simulink model "ex14busSGandPV_sim"  (R2014b)
settings: Solver=ode45  SolverMode=SingleTasking  StartTime=0.0  StopTime=8  MaxStep=0.0008  RelTol=0.0001
values from neighbouring files (symbols this model uses):
  Anf = full(Aksi)    [ex14busSGandPV.m]
  baseV = 1e3*mpcA.bus(1,BASE_KV)    [ex14busSGandPV.m]    (also in ex9busSG_data.mat = 345000; exDroopA.m = 1e3*mpc.bus(:,BASE_KV); exDroopB.m = 1e3*mpc.bus(:,BASE_KV); exLargeSysStability.m = 1e3*mpc.bus(:,BASE_KV))
  Bnf = full(Bksi)    [ex14busSGandPV.m]
  bus1_vd = 2^0.5*1e3    (= 1414.21356237)    [ex3busPV.m]    (also in exLongLinePV.m = 141421.356237)
  Cbus = [600e-6 ; 600e-6]    [ex14busSGandPV.m]    (also in exLongLinePV.m = 0.001)
  Cbus2 = (1e6*mpcC.bus(2,BS))/(ws*baseV^2)    [ex14busSGandPV.m]
  Cbus3 = (1e6*mpcC.bus(3,BS))/(ws*baseV^2)    [ex14busSGandPV.m]
  Cinv = Cinv_pu/(ws*baseZ)    [ex14busSGandPV.m]
  Cnf = full(Cksi)    [ex14busSGandPV.m]
  Dnf = full(Dksi)    [ex14busSGandPV.m]
  If_dc = 0.2*Prt./Ert    [ex14busSGandPV.m]    (also in ex7busLongLine.m = Prt./(60*Vf_dc); exDroopA.m = Prt./(60*Vf_dc); exDroopB.m = Prt./(60*Vf_dc); exSyncGenPVinv.m)
  Kd = KD_GAIN_CNST*J*ws    [ex14busSGandPV.m]    (also in ex2busStability.m = 24000; ex7busLongLine.m; ex9busSG.m; exDroopA.m)
  ki = [0.3 ; 0.3]    [ex14busSGandPV.m]    (also in exLongLinePV.m = 1e-05)
  kp = [1.3e-6 ; 1.3e-6]    [ex14busSGandPV.m]    (also in exLongLinePV.m = 1e-05)
  L0 = 0.1*Ld    [ex14busSGandPV.m]    (also in ex7busLongLine.m; exDroopA.m; exDroopB.m; exSyncGenPVinv.m)
  Laf = (2^0.5)*Ert./(ws*If_dc)    [ex14busSGandPV.m]    (also in ex7busLongLine.m; exDroopA.m; exDroopB.m; exSyncGenPVinv.m = (2^0.5)*5*Ert.^2./(ws*Prt))
  Lb2 = 2*Ld.*Lff - 3*Laf.^2    [ex14busSGandPV.m]    (also in ex7busLongLine.m; exDroopA.m; exDroopB.m; exSyncGenPVinv.m)
  Ld = 0.6*Lpu    [ex14busSGandPV.m]    (also in ex7busLongLine.m = 0.3*Lpu; exDroopA.m = 0.3*Lpu; exDroopB.m = 0.3*Lpu; exSyncGenPVinv.m)
  Lff = 2*Laf.^2./Ld    [ex14busSGandPV.m]    (also in ex7busLongLine.m; exDroopA.m; exDroopB.m; exSyncGenPVinv.m)
  Lq = Ld    [ex14busSGandPV.m]    (also in ex7busLongLine.m; exDroopA.m; exDroopB.m; exSyncGenPVinv.m)
  mpcE = runpf(mpcE)    [ex14busSGandPV.m]    (also in exDroopA.m)
  Nss = length(ssbus)    [ex14busSGandPV.m]
  PG = 2    [ex9busSG_data.mat]
  Pgm = 3*[40; 20]*1e6    [ex14busSGandPV.m]
  poles_2Jws = poles./(2*J*ws)    [ex14busSGandPV.m]    (also in ex2busStability.m = poles./(2*ws*J); ex7busLongLine.m; ex9busSG.m = poles./(2*ws*J); exDroopA.m)
  Pren = [10 ; 10]*1e6    [ex14busSGandPV.m]    (also in ex3busPV.m = 500; exLongLinePV.m = 5000000)
  PT = 16    [ex9busSG_data.mat]
  QG = 3    [ex9busSG_data.mat]
  QT = 17    [ex9busSG_data.mat]
  Ra = 0.05*Ert.^2./Prt    [ex14busSGandPV.m]    (also in ex7busLongLine.m = 0.01*Ert.^2./Prt; exDroopA.m = 0.01*Ert.^2./Prt; exDroopB.m = 0.01*Ert.^2./Prt; exSyncGenPVinv.m)
  Rf = Lff/1.2    [ex14busSGandPV.m]    (also in ex7busLongLine.m = Vf_dc./If_dc; exDroopA.m = Vf_dc./If_dc; exDroopB.m = Vf_dc./If_dc; exSyncGenPVinv.m)
  step_size_bus2 = 0    [ex14busSGandPV.m]
  step_size_bus3 = 0    [ex14busSGandPV.m]
  step_size_bus6 = 0    [ex14busSGandPV.m]
  step_size_bus8 = 0    [ex14busSGandPV.m]
  step_time_bus2 = 3    [ex14busSGandPV.m]
  step_time_bus3 = 3    [ex14busSGandPV.m]
  step_time_bus6 = 5    [ex14busSGandPV.m]
  step_time_bus8 = 5    [ex14busSGandPV.m]
  VA = 9    [ex9busSG_data.mat]
  Vbus_ref = [800 ; 800]    [ex14busSGandPV.m]    (also in exLongLinePV.m = 800)
  Vf_dc = If_dc.*Rf    [ex14busSGandPV.m]    (also in ex7busLongLine.m = 500 * ones(size(Ert)); exDroopA.m = 500 * ones(size(Ert)); exDroopB.m = 500 * ones(size(Ert)); exSyncGenPVinv.m)
  vinf_0 = 0    [ex14busSGandPV.m]    (also in ex7busLongLine.m; exDroopA.m; exSyncGenPVinv.m)
  vinf_d = (2^0.5)*mpcA.bus(1,VM)*baseV    [ex14busSGandPV.m]    (also in ex7busLongLine.m = 250457.221896; exDroopA.m = (2^0.5)*mpc.bus(1,VM)*baseV(1); exSyncGenPVinv.m = (2^0.5)*mpc.bus(1,VM)*baseV(1))
  vinf_q = 0    [ex14busSGandPV.m]    (also in ex7busLongLine.m; exDroopA.m; exSyncGenPVinv.m)
  vinit_dq0_bus2 = [real(vpp) ; imag(vpp) ; 0]    [ex14busSGandPV.m]
  vinit_dq0_bus3 = [real(vpp) ; imag(vpp) ; 0]    [ex14busSGandPV.m]
  vinit_dq0_bus6 = [real(vpp) ; imag(vpp) ; 0]    [ex14busSGandPV.m]
  vinit_dq0_bus8 = [real(vpp) ; imag(vpp) ; 0]    [ex14busSGandPV.m]
  VM = 8    [ex9busSG_data.mat]
  ws = 2*pi*50    (= 314.159265359)    [ex14busSGandPV.m]    (also in ex2busStability.m; ex3busPV.m; ex7busLongLine.m; ex9busSG.m)
libraries: simulink x2
(part 1 of 2)
settings Model: Creator=COPEC  LastModifiedBy=Juri
settings OptimizationCC: BlockReduction=off  BooleanDataType=off
settings DebuggingCC: SaveWithParameterizedLinksMsg=none  UnderspecifiedInitializationDetection=Classic  MergeDetectMultiDrivingBlocksExec=none  SignalResolutionControl=TryResolveAllWithWarning  SolverPrmCheckMsg=none  FrameProcessingCompatibilityMsg=error
settings HardwareCC: TargetUnknown=on

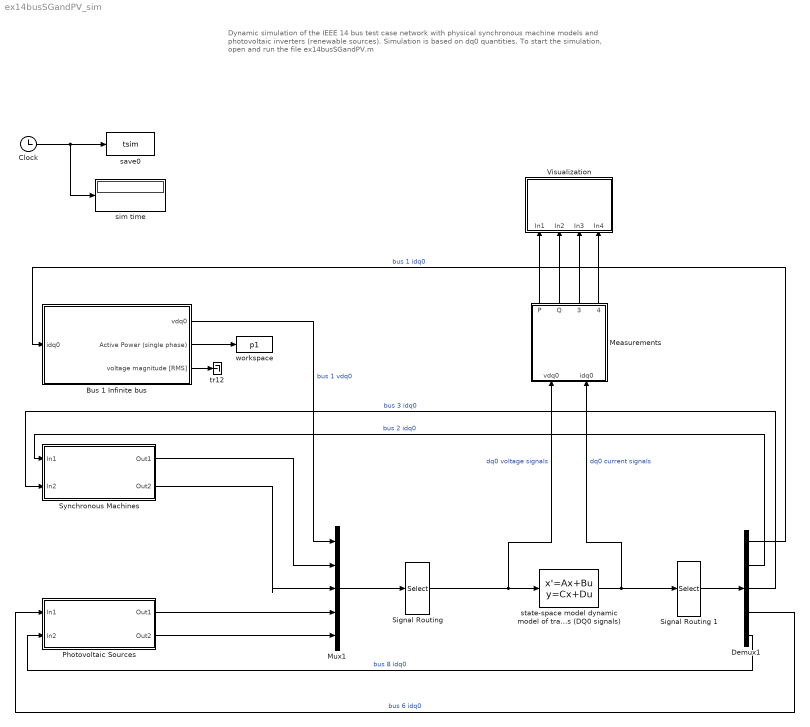
== system ex14busSGandPV_sim ==
  note: Dynamic simulation of the IEEE 14 bus test case network with physical synchronous machine models and photovoltaic inverters (renewable sources). Simulation is based on dq0 quantities.
      |
      | To start the simulation, open and run the file
      | ex14busSGandPV.m
  Bus 1 Infinite bus : Subsystem
  Clock : Clock
  Demux1 : Demux  Outputs=5
  Measurements : Subsystem
  Mux1 : Mux  Inputs=5
  Photovoltaic Sources : Subsystem
  "Signal Routing " : Selector  InputPortWidth=3*Nss  IndexOptions=Index vector (dialog)  Indices=units_to_net  OutputSizes=1
  Signal Routing 1 : Selector  InputPortWidth=3*Nss  IndexOptions=Index vector (dialog)  Indices=net_to_units  OutputSizes=1
  Synchronous Machines : Subsystem
  Visualization : Subsystem
  save0 : ToWorkspace  VariableName=tsim  SampleTime=-1
  sim time : Display
  state-space model dynamic model of transmission network with integrated loads (DQ0 signals) : StateSpace  A=Anf  B=Bnf  C=Cnf  D=Dnf  X0=0
  tr12 : Terminator
  workspace : ToWorkspace  VariableName=p1  SampleTime=-1
  wires:
  Clock/1 -> sim time/1, save0/1
  Mux1/1 -> "Signal Routing "/1
  Signal Routing 1/1 -> Demux1/1
  Bus 1 Infinite bus/3(voltage magnitude [RMS]) -> tr12/1
  Bus 1 Infinite bus/2(Active Power (single phase)) -> workspace/1
  Bus 1 Infinite bus/1(vdq0) -> Mux1/1  "bus 1 vdq0"
  Demux1/1 -> Bus 1 Infinite bus/1(idq0)  "bus 1 idq0"
  "Signal Routing "/1 -> state-space model dynamic model of transmission network with integrated loads (DQ0 signals)/1, Measurements/1(vdq0)  "dq0 voltage signals"
  state-space model dynamic model of transmission network with integrated loads (DQ0 signals)/1 -> Signal Routing 1/1, Measurements/2(idq0)  "dq0 current signals"
  Measurements/1(P) -> Visualization/1(In1)
  Measurements/2(Q) -> Visualization/2(In2)
  Measurements/3(Vm_RMS) -> Visualization/3(In3)
  Measurements/4(Vph_deg) -> Visualization/4(In4)
  Demux1/4 -> Photovoltaic Sources/1(In1)  "bus 6 idq0"
  Demux1/5 -> Photovoltaic Sources/2(In2)  "bus 8 idq0"
  Photovoltaic Sources/1(Out1) -> Mux1/4
  Photovoltaic Sources/2(Out2) -> Mux1/5
  Demux1/2 -> Synchronous Machines/1(In1)  "bus 2 idq0"
  Demux1/3 -> Synchronous Machines/2(In2)  "bus 3 idq0"
  Synchronous Machines/1(Out1) -> Mux1/2
  Synchronous Machines/2(Out2) -> Mux1/3

== system ex14busSGandPV_sim/Bus 1 Infinite bus ==
  idq0 : Inport
  Constant : Constant  Value=vinf_d
  Constant1 : Constant  Value=vinf_q
  Constant2 : Constant  Value=vinf_0
  Mux1 : Mux  Inputs=3
  Terminator1 : Terminator
  Terminator2 : Terminator
  measurements : Subsystem
  vdq0 : Outport
  Active Power (single phase) : Outport  Port=2
  voltage magnitude [RMS] : Outport  Port=3
  wires:
  measurements/1(P) -> Active Power (single phase)/1
  measurements/2(Q) -> Terminator1/1
  measurements/3(Vm_RMS) -> voltage magnitude [RMS]/1
  measurements/4(Vph_deg) -> Terminator2/1
  idq0/1 -> measurements/2(idq0)
  Mux1/1 -> measurements/1(vdq0), vdq0/1
  Constant/1 -> Mux1/1
  Constant1/1 -> Mux1/2
  Constant2/1 -> Mux1/3

== system ex14busSGandPV_sim/Measurements ==
  vdq0 : Inport
  idq0 : Inport  Port=2
  Add : Sum  Inputs=+++
  Add1 : Sum  Inputs=+-
  Add2 : Sum
  Demux : Demux  Outputs=3
  Demux1 : Demux  Outputs=3
  Gain : Gain  Gain=0.5
  Gain1 : Gain  Gain=0.5
  Gain2 : Gain  Gain=0.5
  Gain3 : Gain  Gain=2
  Gain4 : Gain  Gain=180/pi
  Math Function : Math  Operator=square  SaturateOnIntegerOverflow=on
  Math Function1 : Math  Operator=square  SaturateOnIntegerOverflow=on
  Sqrt : Sqrt  SaturateOnIntegerOverflow=on
  Trigonometric Function : Trigonometry  Operator=atan2
  mult{,1..4} (5 alike) : Product  Inputs=**
  P : Outport
  Q : Outport  Port=2
  Vm_RMS : Outport  Port=3
  Vph_deg : Outport  Port=4
  wires:
  idq0/1 -> Demux1/1
  vdq0/1 -> Demux/1
  Demux/1 -> Math Function/1, Trigonometric Function/2, mult3/1, mult/1  "vd"
  Demux/2 -> Trigonometric Function/1, Math Function1/1, mult2/1, mult1/1  "vq"
  Demux1/1 -> mult/2, mult2/2  "id"
  Demux1/2 -> mult3/2, mult1/2  "iq"
  Demux/3 -> mult4/1  "v0"
  Demux1/3 -> mult4/2  "i0"
  mult/1 -> Add/1
  mult1/1 -> Add/2
  Add/1 -> Gain/1
  mult2/1 -> Add1/1
  mult3/1 -> Add1/2
  Add1/1 -> Gain1/1
  Sqrt/1 -> Vm_RMS/1
  Math Function/1 -> Add2/1
  Math Function1/1 -> Add2/2
  Add2/1 -> Gain2/1
  Gain2/1 -> Sqrt/1
  Gain/1 -> P/1
  Gain1/1 -> Q/1
  mult4/1 -> Gain3/1
  Gain3/1 -> Add/3
  Trigonometric Function/1 -> Gain4/1
  Gain4/1 -> Vph_deg/1

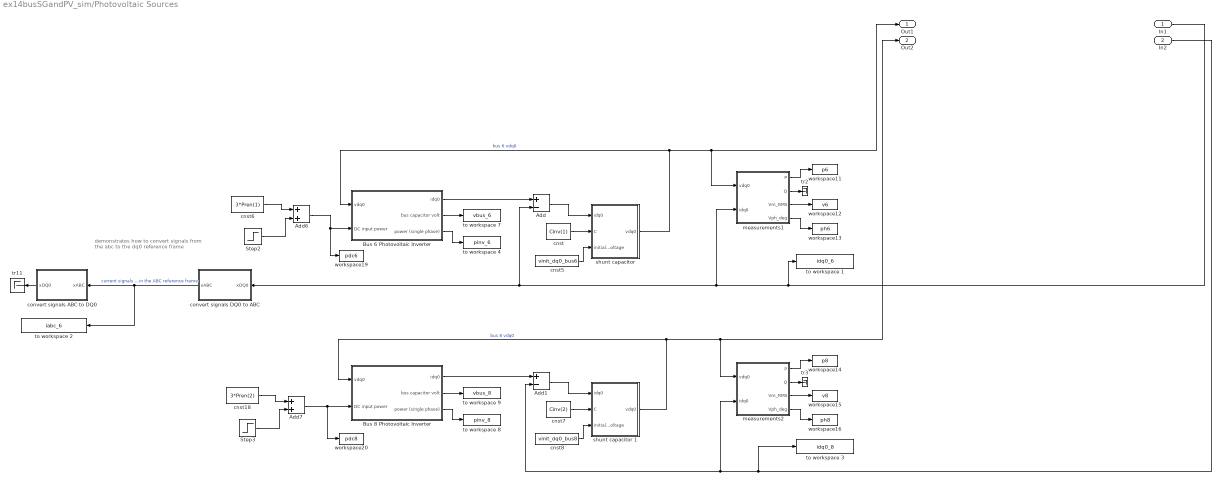
== system ex14busSGandPV_sim/Photovoltaic Sources ==
  note: demonstrates how to convert signals
      | from the abc to the dq0 reference frame
  In1 : Inport
  In2 : Inport  Port=2
  Add : Sum  Inputs=+-
  Add1 : Sum  Inputs=+-
  Add6 : Sum
  Add7 : Sum
  Bus 6 Photovoltaic Inverter : Subsystem
  Bus 8 Photovoltaic Inverter : Subsystem
  Step2 : Step  Time=step_time_bus6  After=step_size_bus6  SampleTime=0
  Step3 : Step  Time=step_time_bus8  After=step_size_bus8  SampleTime=0
  cnst : Constant  Value=Cinv(1)
  cnst18 : Constant  Value=3*Pren(2)
  cnst5 : Constant  Value=vinit_dq0_bus6
  cnst6 : Constant  Value=3*Pren(1)
  cnst7 : Constant  Value=Cinv(2)
  cnst8 : Constant  Value=vinit_dq0_bus8
  convert signals ABC to DQ0 : Subsystem
  convert signals DQ0 to ABC : Subsystem
  measurements1 : Subsystem
  measurements2 : Subsystem
  shunt capacitor : Subsystem
  shunt capacitor 1 : Subsystem
  to workspace 1 : ToWorkspace  VariableName=idq0_6  SampleTime=-1
  to workspace 2 : ToWorkspace  VariableName=iabc_6  SampleTime=-1
  to workspace 3 : ToWorkspace  VariableName=idq0_8  SampleTime=-1
  to workspace 4 : ToWorkspace  VariableName=pinv_6  SampleTime=-1
  to workspace 7 : ToWorkspace  VariableName=vbus_6  SampleTime=-1
  to workspace 8 : ToWorkspace  VariableName=pinv_8  SampleTime=-1
  to workspace 9 : ToWorkspace  VariableName=vbus_8  SampleTime=-1
  tr11 : Terminator
  tr2 : Terminator
  tr3 : Terminator
  workspace11 : ToWorkspace  VariableName=p6  SampleTime=-1
  workspace12 : ToWorkspace  VariableName=v6  SampleTime=-1
  workspace13 : ToWorkspace  VariableName=ph6  SampleTime=-1
  workspace14 : ToWorkspace  VariableName=p8  SampleTime=-1
  workspace15 : ToWorkspace  VariableName=v8  SampleTime=-1
  workspace16 : ToWorkspace  VariableName=ph8  SampleTime=-1
  workspace19 : ToWorkspace  VariableName=pdc6  SampleTime=-1
  workspace20 : ToWorkspace  VariableName=pdc8  SampleTime=-1
  Out1 : Outport
  Out2 : Outport  Port=2
  wires:
  shunt capacitor/1(vdq0) -> Out1/1, measurements1/1(vdq0), Bus 6 Photovoltaic Inverter/1(vdq0)  "bus 6 vdq0"
  Add/1 -> shunt capacitor/1(idq0)
  cnst/1 -> shunt capacitor/2(C)
  convert signals ABC to DQ0/1(xDQ0) -> tr11/1
  convert signals DQ0 to ABC/1(xABC) -> convert signals ABC to DQ0/1(xABC), to workspace 2/1  "current signals in the ABC reference frame"
  Bus 6 Photovoltaic Inverter/1(idq0) -> Add/1
  In1/1 -> convert signals DQ0 to ABC/1(xDQ0), Add/2, measurements1/2(idq0), to workspace 1/1
  Add1/1 -> shunt capacitor 1/1(idq0)
  cnst7/1 -> shunt capacitor 1/2(C)
  Bus 8 Photovoltaic Inverter/1(idq0) -> Add1/1
  cnst5/1 -> shunt capacitor/3(initial voltage)
  Add7/1 -> workspace20/1, Bus 8 Photovoltaic Inverter/2(DC input power)
  shunt capacitor 1/1(vdq0) -> Bus 8 Photovoltaic Inverter/1(vdq0), Out2/1, measurements2/1(vdq0)  "bus 8 vdq0"
  Add6/1 -> workspace19/1, Bus 6 Photovoltaic Inverter/2(DC input power)
  cnst8/1 -> shunt capacitor 1/3(initial voltage)
  measurements1/2(Q) -> tr2/1
  measurements1/1(P) -> workspace11/1
  measurements1/3(Vm_RMS) -> workspace12/1
  In2/1 -> to workspace 3/1, measurements2/2(idq0), Add1/2
  measurements2/2(Q) -> tr3/1
  measurements2/1(P) -> workspace14/1
  measurements2/3(Vm_RMS) -> workspace15/1
  measurements2/4(Vph_deg) -> workspace16/1
  measurements1/4(Vph_deg) -> workspace13/1
  Step3/1 -> Add7/2
  cnst6/1 -> Add6/1
  cnst18/1 -> Add7/1
  Bus 8 Photovoltaic Inverter/2(bus capacitor volt) -> to workspace 9/1
  Bus 6 Photovoltaic Inverter/3(power (single phase)) -> to workspace 4/1
  Bus 8 Photovoltaic Inverter/3(power (single phase)) -> to workspace 8/1
  Step2/1 -> Add6/2
  Bus 6 Photovoltaic Inverter/2(bus capacitor volt) -> to workspace 7/1

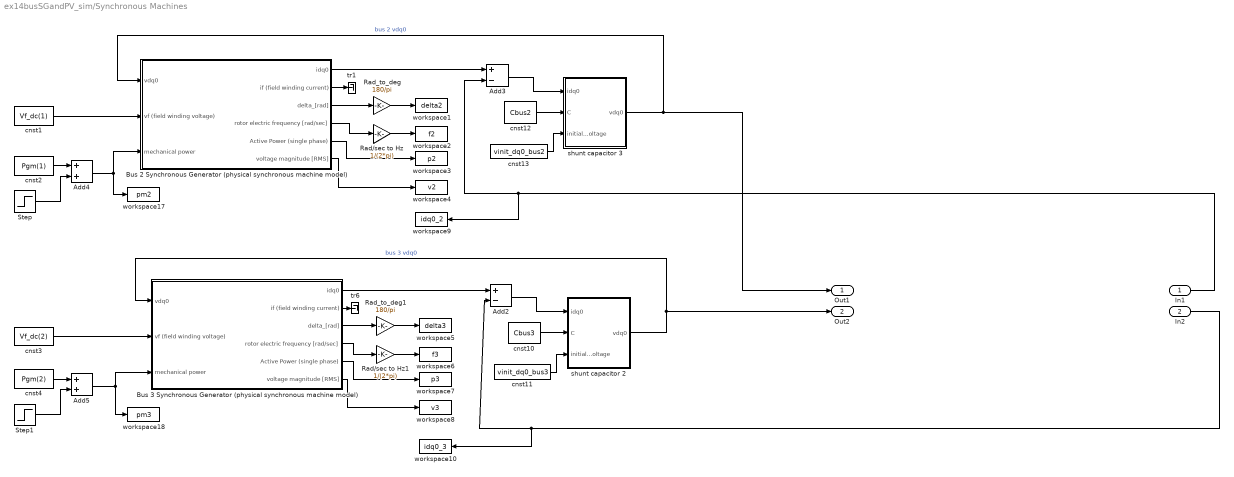
== system ex14busSGandPV_sim/Synchronous Machines ==
  In1 : Inport
  In2 : Inport  Port=2
  Add2 : Sum  Inputs=+-
  Add3 : Sum  Inputs=+-
  Add4 : Sum
  Add5 : Sum
  Bus 2 Synchronous Generator (physical synchronous machine model) : Subsystem
  Bus 3 Synchronous Generator (physical synchronous machine model) : Subsystem
  Rad/sec to Hz : Gain  Gain=1/(2*pi)
  Rad/sec to Hz1 : Gain  Gain=1/(2*pi)
  Rad_to_deg : Gain  Gain=180/pi
  Rad_to_deg1 : Gain  Gain=180/pi
  Step : Step  Time=step_time_bus2  After=step_size_bus2  SampleTime=0
  Step1 : Step  Time=step_time_bus3  After=step_size_bus3  SampleTime=0
  cnst1 : Constant  Value=Vf_dc(1)
  cnst10 : Constant  Value=Cbus3
  cnst11 : Constant  Value=vinit_dq0_bus3
  cnst12 : Constant  Value=Cbus2
  cnst13 : Constant  Value=vinit_dq0_bus2
  cnst2 : Constant  Value=Pgm(1)
  cnst3 : Constant  Value=Vf_dc(2)
  cnst4 : Constant  Value=Pgm(2)
  shunt capacitor 2 : Subsystem
  shunt capacitor 3 : Subsystem
  tr1 : Terminator
  tr6 : Terminator
  workspace1 : ToWorkspace  VariableName=delta2  SampleTime=-1
  workspace10 : ToWorkspace  VariableName=idq0_3  SampleTime=-1
  workspace17 : ToWorkspace  VariableName=pm2  SampleTime=-1
  workspace18 : ToWorkspace  VariableName=pm3  SampleTime=-1
  workspace2 : ToWorkspace  VariableName=f2  SampleTime=-1
  workspace3 : ToWorkspace  VariableName=p2  SampleTime=-1
  workspace4 : ToWorkspace  VariableName=v2  SampleTime=-1
  workspace5 : ToWorkspace  VariableName=delta3  SampleTime=-1
  workspace6 : ToWorkspace  VariableName=f3  SampleTime=-1
  workspace7 : ToWorkspace  VariableName=p3  SampleTime=-1
  workspace8 : ToWorkspace  VariableName=v3  SampleTime=-1
  workspace9 : ToWorkspace  VariableName=idq0_2  SampleTime=-1
  Out1 : Outport
  Out2 : Outport  Port=2
  wires:
  shunt capacitor 2/1(vdq0) -> Out2/1, Bus 3 Synchronous Generator (physical synchronous machine model)/1(vdq0)  "bus 3 vdq0"
  cnst11/1 -> shunt capacitor 2/3(initial voltage)
  cnst13/1 -> shunt capacitor 3/3(initial voltage)
  In2/1 -> workspace10/1, Add2/2
  Bus 2 Synchronous Generator (physical synchronous machine model)/1(idq0) -> Add3/1
  cnst12/1 -> shunt capacitor 3/2(C)
  Add2/1 -> shunt capacitor 2/1(idq0)
  Add3/1 -> shunt capacitor 3/1(idq0)
  shunt capacitor 3/1(vdq0) -> Out1/1, Bus 2 Synchronous Generator (physical synchronous machine model)/1(vdq0)  "bus 2 vdq0"
  cnst10/1 -> shunt capacitor 2/2(C)
  In1/1 -> Add3/2, workspace9/1
  Bus 3 Synchronous Generator (physical synchronous machine model)/1(idq0) -> Add2/1
  Bus 3 Synchronous Generator (physical synchronous machine model)/6(voltage magnitude [RMS]) -> workspace8/1
  Bus 2 Synchronous Generator (physical synchronous machine model)/3(delta_[rad]) -> Rad_to_deg/1
  Bus 3 Synchronous Generator (physical synchronous machine model)/5(Active Power (single phase)) -> workspace7/1
  cnst3/1 -> Bus 3 Synchronous Generator (physical synchronous machine model)/2(vf (field winding voltage))
  Bus 2 Synchronous Generator (physical synchronous machine model)/4(rotor electric frequency [rad/sec]) -> Rad/sec to Hz/1
  Bus 3 Synchronous Generator (physical synchronous machine model)/2(if (field winding current)) -> tr6/1
  Bus 3 Synchronous Generator (physical synchronous machine model)/4(rotor electric frequency [rad/sec]) -> Rad/sec to Hz1/1
  cnst1/1 -> Bus 2 Synchronous Generator (physical synchronous machine model)/2(vf (field winding voltage))
  Rad_to_deg/1 -> workspace1/1
  Rad_to_deg1/1 -> workspace5/1
  Bus 3 Synchronous Generator (physical synchronous machine model)/3(delta_[rad]) -> Rad_to_deg1/1
  Rad/sec to Hz/1 -> workspace2/1
  Rad/sec to Hz1/1 -> workspace6/1
  Bus 2 Synchronous Generator (physical synchronous machine model)/5(Active Power (single phase)) -> workspace3/1
  Add5/1 -> workspace18/1, Bus 3 Synchronous Generator (physical synchronous machine model)/3(mechanical power)
  Bus 2 Synchronous Generator (physical synchronous machine model)/6(voltage magnitude [RMS]) -> workspace4/1
  Bus 2 Synchronous Generator (physical synchronous machine model)/2(if (field winding current)) -> tr1/1
  Add4/1 -> workspace17/1, Bus 2 Synchronous Generator (physical synchronous machine model)/3(mechanical power)
  cnst4/1 -> Add5/1
  Step/1 -> Add4/2
  Step1/1 -> Add5/2
  cnst2/1 -> Add4/1

== system ex14busSGandPV_sim/Visualization ==
  note: equal to steady-state solution
      | with no step in inputs
  note: network measurements
  note: power flow
      | solution
      | (steady-state)
  In1 : Inport
  In2 : Inport  Port=2
  In3 : Inport  Port=3
  In4 : Inport  Port=4
  Gain6 : Gain  Gain=1e-6
  Gain7 : Gain  Gain=1e-6
  Gain8 : Gain  Gain=1e-3
  active power 1  [MW] : Display
  active power 2  [MW] : Display
  cnst14 : Constant  Value=mpcE.bus([1 2 3 6 8],VM)*baseV/1e3
  cnst15 : Constant  Value=mpcE.bus([1 2 3 6 8],VA)
  cnst16 : Constant  Value=[mpcE.gen(1,PG); -mpcE.branch([21 22],PT); Pren/1e6]
  cnst17 : Constant  Value=[mpcE.gen(1,QG); -mpcE.branch([21 22],QT)+((baseV^2)*ws/1e6)*mpcE.bus([2,3],VM).^2.*[Cbus2;Cbus3]; ((baseV^2)*ws/1e6)*mpcE.bus([6,8],VM).^2.*Cinv]
  reactive power 1 [MVAr] : Display
  reactive power 2  [MVAr] : Display
  to workspace 5 : ToWorkspace  VariableName=netp  SampleTime=-1
  to workspace 6 : ToWorkspace  VariableName=netq  SampleTime=-1
  "voltage amplitudes 1  kV RMS " : Display
  voltage amplitudes 2  kV RMS : Display
  voltage phases 1 [deg] : Display
  voltage phases 2 [deg] : Display
  wires:
  Gain6/1 -> active power 1  [MW]/1, to workspace 5/1
  Gain8/1 -> "voltage amplitudes 1  kV RMS "/1
  In3/1 -> Gain8/1
  In1/1 -> Gain6/1
  In2/1 -> Gain7/1
  In4/1 -> voltage phases 1 [deg]/1
  Gain7/1 -> reactive power 1 [MVAr]/1, to workspace 6/1
  cnst14/1 -> voltage amplitudes 2  kV RMS/1
  cnst16/1 -> active power 2  [MW]/1
  cnst17/1 -> reactive power 2  [MVAr]/1
  cnst15/1 -> voltage phases 2 [deg]/1

== system ex14busSGandPV_sim/Bus 1 Infinite bus/measurements ==
  vdq0 : Inport
  idq0 : Inport  Port=2
  Add : Sum  Inputs=+++
  Add1 : Sum  Inputs=+-
  Add2 : Sum
  Demux : Demux  Outputs=3
  Demux1 : Demux  Outputs=3
  Gain : Gain  Gain=0.5
  Gain1 : Gain  Gain=0.5
  Gain2 : Gain  Gain=0.5
  Gain3 : Gain  Gain=2
  Gain4 : Gain  Gain=180/pi
  Math Function : Math  Operator=square  SaturateOnIntegerOverflow=on
  Math Function1 : Math  Operator=square  SaturateOnIntegerOverflow=on
  Sqrt : Sqrt  SaturateOnIntegerOverflow=on
  Trigonometric Function : Trigonometry  Operator=atan2
  mult{,1..4} (5 alike) : Product  Inputs=**
  P : Outport
  Q : Outport  Port=2
  Vm_RMS : Outport  Port=3
  Vph_deg : Outport  Port=4
  wires:
  idq0/1 -> Demux1/1
  vdq0/1 -> Demux/1
  Demux/1 -> Math Function/1, Trigonometric Function/2, mult3/1, mult/1  "vd"
  Demux/2 -> Trigonometric Function/1, Math Function1/1, mult2/1, mult1/1  "vq"
  Demux1/1 -> mult/2, mult2/2  "id"
  Demux1/2 -> mult3/2, mult1/2  "iq"
  Demux/3 -> mult4/1  "v0"
  Demux1/3 -> mult4/2  "i0"
  mult/1 -> Add/1
  mult1/1 -> Add/2
  Add/1 -> Gain/1
  mult2/1 -> Add1/1
  mult3/1 -> Add1/2
  Add1/1 -> Gain1/1
  Sqrt/1 -> Vm_RMS/1
  Math Function/1 -> Add2/1
  Math Function1/1 -> Add2/2
  Add2/1 -> Gain2/1
  Gain2/1 -> Sqrt/1
  Gain/1 -> P/1
  Gain1/1 -> Q/1
  mult4/1 -> Gain3/1
  Gain3/1 -> Add/3
  Trigonometric Function/1 -> Gain4/1
  Gain4/1 -> Vph_deg/1

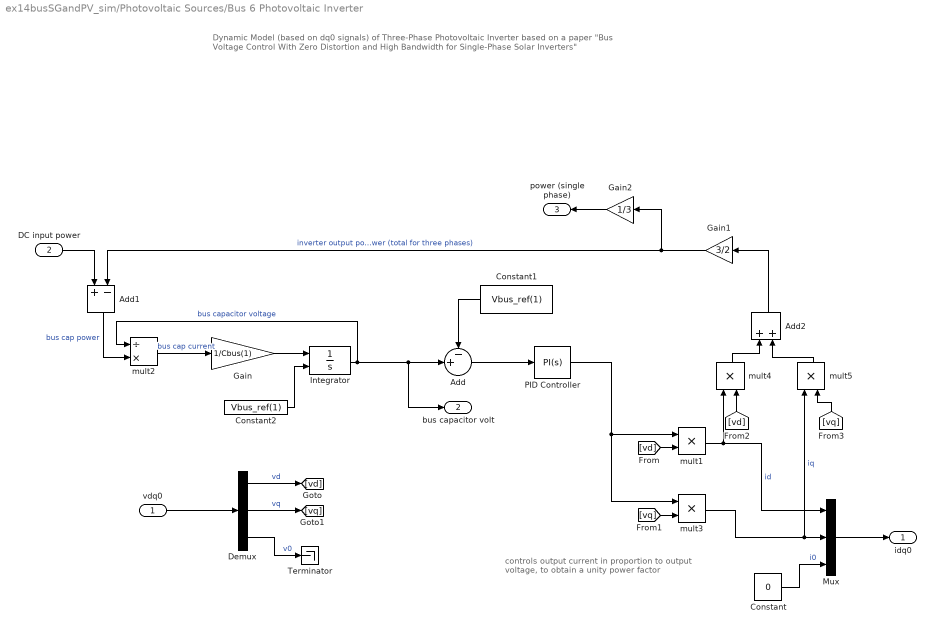
== system ex14busSGandPV_sim/Photovoltaic Sources/Bus 6 Photovoltaic Inverter ==
  note: controls output current in proportion
      | to output voltage, to obtain a unity power factor
  note: Dynamic Model (based on dq0 signals)
      | of Three-Phase Photovoltaic Inverter
      |
      | based on a paper "Bus Voltage Control With Zero
      | Distortion and High Bandwidth for Single-Phase Solar Inverters"
  vdq0 : Inport
  DC input power : Inport  Port=2
  Add : Sum  Inputs=-+|
  Add1 : Sum  Inputs=+-
  Add2 : Sum
  Constant : Constant  Value=0
  Constant1 : Constant  Value=Vbus_ref(1)
  Constant2 : Constant  Value=Vbus_ref(1)
  Demux : Demux  Outputs=3
  Gain : Gain  Gain=1/Cbus(1)
  Gain1 : Gain  Gain=3/2
  Gain2 : Gain  Gain=1/3
  Integrator : Integrator  InitialConditionSource=external  InitialCondition=Vbus_ref(1)*0.8  LowerSaturationLimit=50
  Mux : Mux  Inputs=3
  PID Controller : simulink/Continuous/PID Controller  Controller=PI  TimeDomain=Continuous-time  SampleTime=-1  IntegratorMethod=Forward Euler  FilterMethod=Forward Euler  Form=Parallel  UseFilter=on  ControllerParametersSource=internal  P=kp(1)  I=ki(1)  D=0  N=100  InitialConditionSource=internal  InitialConditionForIntegrator=0  InitialConditionForFilter=0  ExternalReset=none  LimitOutput=off  UpperSaturationLimit=inf  LowerSaturationLimit=-inf  LinearizeAsGain=on  AntiWindupMode=none  Kb=1  TrackingMode=off  Kt=1  PParamMin=[]  PParamMax=[]  IParamMin=[]  IParamMax=[]  DParamMin=[]  DParamMax=[]  NParamMin=[]  NParamMax=[]  KbParamMin=[]  KbParamMax=[]  KtParamMin=[]  KtParamMax=[]  POutMin=[]  POutMax=[]  IOutMin=[]  IOutMax=[]  DOutMin=[]  DOutMax=[]  NOutMin=[]  NOutMax=[]  KbOutMin=[]  KbOutMax=[]  KtOutMin=[]  KtOutMax=[]  IntegratorOutMin=[]  IntegratorOutMax=[]  FilterOutMin=[]  FilterOutMax=[]  SumOutMin=[]  SumOutMax=[]  SumI1OutMin=[]  SumI1OutMax=[]  SumI2OutMin=[]  SumI2OutMax=[]  SumI3OutMin=[]  SumI3OutMax=[]  SumDOutMin=[]  SumDOutMax=[]  SaturationOutMin=[]  SaturationOutMax=[]  IntegratorContinuousStateAttributes=''  IntegratorStateMustResolveToSignalObject=off  IntegratorRTWStateStorageClass=Auto  FilterContinuousStateAttributes=''  FilterStateMustResolveToSignalObject=off  FilterRTWStateStorageClass=Auto  DifferentiatorICPrevScaledInput=0  DifferentiatorOutMin=[]  DifferentiatorOutMax=[]
  Terminator : Terminator
  mult{1,3..5} (4 alike) : Product  Inputs=**
  mult2 : Product  Inputs=/*
  idq0 : Outport
  bus capacitor volt : Outport  Port=2
  power (single phase) : Outport  Port=3
  wires:
  vdq0/1 -> Demux/1
  Demux/3 -> Terminator/1  "v0"
  Mux/1 -> idq0/1
  mult1/1 -> mult4/1, Mux/1  "id"
  mult3/1 -> mult5/1, Mux/2  "iq"
  Constant/1 -> Mux/3  "i0"
  Demux/1 -> [vd]  "vd"
  Demux/2 -> [vq]  "vq"
  PID Controller/1 -> mult1/1, mult3/1
  Add/1 -> PID Controller/1
  Constant1/1 -> Add/1
  Integrator/1 -> mult2/1, bus capacitor volt/1, Add/2  "bus capacitor voltage"
  mult2/1 -> Gain/1  "bus cap current"
  Gain/1 -> Integrator/1
  Add1/1 -> mult2/2  "bus cap power"
  DC input power/1 -> Add1/1
  Gain1/1 -> Gain2/1, Add1/2  "inverter output power (total for three phases)"
  [vd] -> mult1/2
  [vq] -> mult3/2
  [vd] -> mult4/2
  [vq] -> mult5/2
  mult4/1 -> Add2/1
  mult5/1 -> Add2/2
  Add2/1 -> Gain1/1
  Constant2/1 -> Integrator/2
  Gain2/1 -> power (single phase)/1

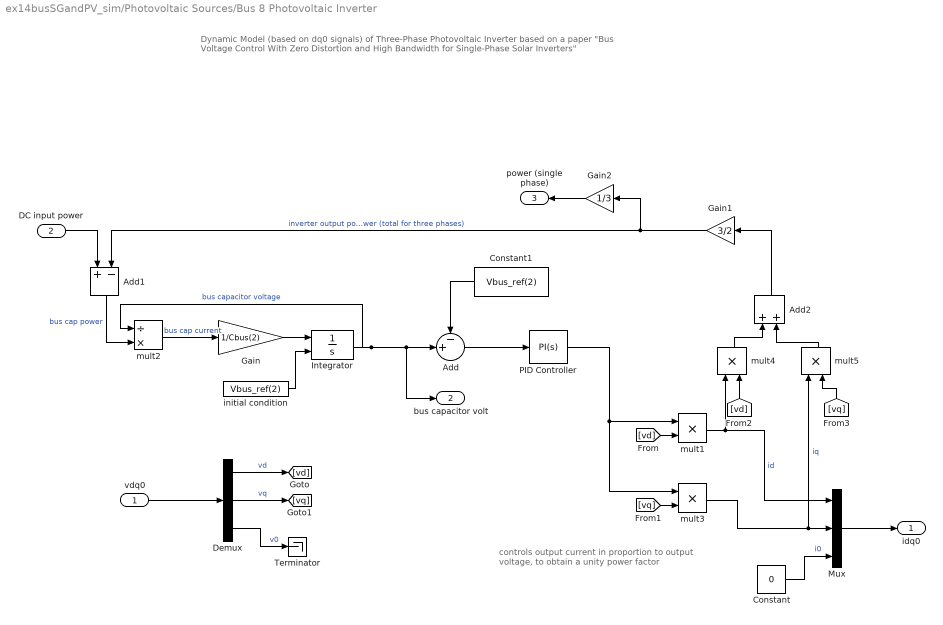
== system ex14busSGandPV_sim/Photovoltaic Sources/Bus 8 Photovoltaic Inverter ==
  note: controls output current in proportion
      | to output voltage, to obtain a unity power factor
  note: Dynamic Model (based on dq0 signals)
      | of Three-Phase Photovoltaic Inverter
      |
      | based on a paper "Bus Voltage Control With Zero
      | Distortion and High Bandwidth for Single-Phase Solar Inverters"
  vdq0 : Inport
  DC input power : Inport  Port=2
  Add : Sum  Inputs=-+|
  Add1 : Sum  Inputs=+-
  Add2 : Sum
  Constant : Constant  Value=0
  Constant1 : Constant  Value=Vbus_ref(2)
  Demux : Demux  Outputs=3
  Gain : Gain  Gain=1/Cbus(2)
  Gain1 : Gain  Gain=3/2
  Gain2 : Gain  Gain=1/3
  Integrator : Integrator  InitialConditionSource=external  InitialCondition=Vbus_ref(1)*0.8  LowerSaturationLimit=50
  Mux : Mux  Inputs=3
  PID Controller : simulink/Continuous/PID Controller  Controller=PI  TimeDomain=Continuous-time  SampleTime=-1  IntegratorMethod=Forward Euler  FilterMethod=Forward Euler  Form=Parallel  UseFilter=on  ControllerParametersSource=internal  P=kp(2)  I=ki(2)  D=0  N=100  InitialConditionSource=internal  InitialConditionForIntegrator=0  InitialConditionForFilter=0  ExternalReset=none  LimitOutput=off  UpperSaturationLimit=inf  LowerSaturationLimit=-inf  LinearizeAsGain=on  AntiWindupMode=none  Kb=1  TrackingMode=off  Kt=1  PParamMin=[]  PParamMax=[]  IParamMin=[]  IParamMax=[]  DParamMin=[]  DParamMax=[]  NParamMin=[]  NParamMax=[]  KbParamMin=[]  KbParamMax=[]  KtParamMin=[]  KtParamMax=[]  POutMin=[]  POutMax=[]  IOutMin=[]  IOutMax=[]  DOutMin=[]  DOutMax=[]  NOutMin=[]  NOutMax=[]  KbOutMin=[]  KbOutMax=[]  KtOutMin=[]  KtOutMax=[]  IntegratorOutMin=[]  IntegratorOutMax=[]  FilterOutMin=[]  FilterOutMax=[]  SumOutMin=[]  SumOutMax=[]  SumI1OutMin=[]  SumI1OutMax=[]  SumI2OutMin=[]  SumI2OutMax=[]  SumI3OutMin=[]  SumI3OutMax=[]  SumDOutMin=[]  SumDOutMax=[]  SaturationOutMin=[]  SaturationOutMax=[]  IntegratorContinuousStateAttributes=''  IntegratorStateMustResolveToSignalObject=off  IntegratorRTWStateStorageClass=Auto  FilterContinuousStateAttributes=''  FilterStateMustResolveToSignalObject=off  FilterRTWStateStorageClass=Auto  DifferentiatorICPrevScaledInput=0  DifferentiatorOutMin=[]  DifferentiatorOutMax=[]
  Terminator : Terminator
  initial condition : Constant  Value=Vbus_ref(2)
  mult{1,3..5} (4 alike) : Product  Inputs=**
  mult2 : Product  Inputs=/*
  idq0 : Outport
  bus capacitor volt : Outport  Port=2
  power (single phase) : Outport  Port=3
  wires:
  vdq0/1 -> Demux/1
  Demux/3 -> Terminator/1  "v0"
  Mux/1 -> idq0/1
  mult1/1 -> mult4/1, Mux/1  "id"
  mult3/1 -> mult5/1, Mux/2  "iq"
  Constant/1 -> Mux/3  "i0"
  Demux/1 -> [vd]  "vd"
  Demux/2 -> [vq]  "vq"
  PID Controller/1 -> mult1/1, mult3/1
  Add/1 -> PID Controller/1
  Constant1/1 -> Add/1
  Integrator/1 -> mult2/1, bus capacitor volt/1, Add/2  "bus capacitor voltage"
  mult2/1 -> Gain/1  "bus cap current"
  Gain/1 -> Integrator/1
  Add1/1 -> mult2/2  "bus cap power"
  DC input power/1 -> Add1/1
  Gain1/1 -> Gain2/1, Add1/2  "inverter output power (total for three phases)"
  [vd] -> mult1/2
  [vq] -> mult3/2
  [vd] -> mult4/2
  [vq] -> mult5/2
  mult4/1 -> Add2/1
  mult5/1 -> Add2/2
  Add2/1 -> Gain1/1
  initial condition/1 -> Integrator/2
  Gain2/1 -> power (single phase)/1

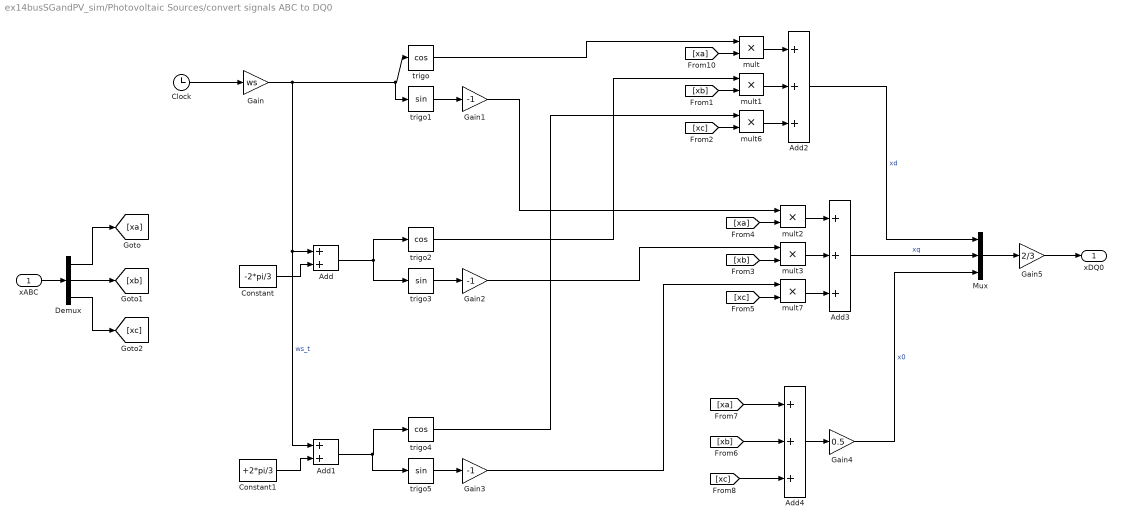
== system ex14busSGandPV_sim/Photovoltaic Sources/convert signals ABC to DQ0 ==
  xABC : Inport
  Add : Sum
  Add1 : Sum
  Add2 : Sum  Inputs=+++
  Add3 : Sum  Inputs=+++
  Add4 : Sum  Inputs=+++
  Clock : Clock
  Constant : Constant  Value=-2*pi/3
  Constant1 : Constant  Value=+2*pi/3
  Demux : Demux  Outputs=3
  Gain : Gain  Gain=ws
  Gain1 : Gain  Gain=-1
  Gain2 : Gain  Gain=-1
  Gain3 : Gain  Gain=-1
  Gain4 : Gain  Gain=0.5
  Gain5 : Gain  Gain=2/3
  Mux : Mux  Inputs=3
  mult{,1..3,6..7} (6 alike) : Product  Inputs=**
  trigo : Trigonometry  Operator=cos
  trigo1 : Trigonometry
  trigo2 : Trigonometry  Operator=cos
  trigo3 : Trigonometry
  trigo4 : Trigonometry  Operator=cos
  trigo5 : Trigonometry
  xDQ0 : Outport
  wires:
  Gain5/1 -> xDQ0/1
  Mux/1 -> Gain5/1
  Gain3/1 -> mult7/1
  Gain2/1 -> mult3/1
  Gain1/1 -> mult2/1
  [xc] -> Add4/3
  [xb] -> Add4/2
  [xa] -> Add4/1
  Add4/1 -> Gain4/1
  mult7/1 -> Add3/3
  [xc] -> mult7/2
  [xb] -> mult3/2
  [xa] -> mult2/2
  trigo4/1 -> mult6/1
  mult6/1 -> Add2/3
  [xc] -> mult6/2
  trigo2/1 -> mult1/1
  trigo/1 -> mult/1
  Gain4/1 -> Mux/3  "x0"
  Add3/1 -> Mux/2  "xq"
  Add2/1 -> Mux/1  "xd"
  mult3/1 -> Add3/2
  mult2/1 -> Add3/1
  [xb] -> mult1/2
  [xa] -> mult/2
  mult1/1 -> Add2/2
  mult/1 -> Add2/1
  Demux/3 -> [xc]
  Demux/2 -> [xb]
  Demux/1 -> [xa]
  xABC/1 -> Demux/1
  Add1/1 -> trigo4/1, trigo5/1
  trigo5/1 -> Gain3/1
  Add/1 -> trigo3/1, trigo2/1
  trigo3/1 -> Gain2/1
  trigo1/1 -> Gain1/1
  Constant1/1 -> Add1/2
  Constant/1 -> Add/2
  Gain/1 -> Add/1, Add1/1, trigo/1, trigo1/1  "ws_t"
  Clock/1 -> Gain/1

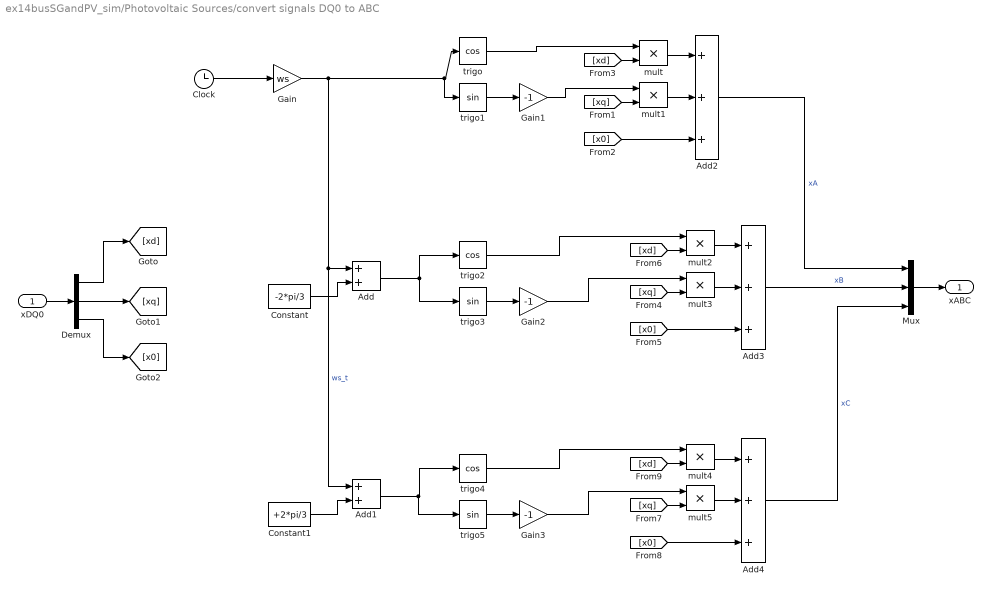
== system ex14busSGandPV_sim/Photovoltaic Sources/convert signals DQ0 to ABC ==
  xDQ0 : Inport
  Add : Sum
  Add1 : Sum
  Add2 : Sum  Inputs=+++
  Add3 : Sum  Inputs=+++
  Add4 : Sum  Inputs=+++
  Clock : Clock
  Constant : Constant  Value=-2*pi/3
  Constant1 : Constant  Value=+2*pi/3
  Demux : Demux  Outputs=3
  Gain : Gain  Gain=ws
  Gain1 : Gain  Gain=-1
  Gain2 : Gain  Gain=-1
  Gain3 : Gain  Gain=-1
  Mux : Mux  Inputs=3
  mult{,1..5} (6 alike) : Product  Inputs=**
  trigo : Trigonometry  Operator=cos
  trigo1 : Trigonometry
  trigo2 : Trigonometry  Operator=cos
  trigo3 : Trigonometry
  trigo4 : Trigonometry  Operator=cos
  trigo5 : Trigonometry
  xABC : Outport
  wires:
  Clock/1 -> Gain/1
  Gain/1 -> trigo1/1, trigo/1, Add1/1, Add/1  "ws_t"
  Constant/1 -> Add/2
  Constant1/1 -> Add1/2
  trigo1/1 -> Gain1/1
  trigo3/1 -> Gain2/1
  Add/1 -> trigo2/1, trigo3/1
  trigo5/1 -> Gain3/1
  Add1/1 -> trigo5/1, trigo4/1
  xDQ0/1 -> Demux/1
  Demux/1 -> [xd]
  Demux/2 -> [xq]
  Demux/3 -> [x0]
  Mux/1 -> xABC/1
  mult/1 -> Add2/1
  mult1/1 -> Add2/2
  [xd] -> mult/2
  [xq] -> mult1/2
  [x0] -> Add2/3
  mult2/1 -> Add3/1
  mult3/1 -> Add3/2
  [xd] -> mult2/2
  [xq] -> mult3/2
  [x0] -> Add3/3
  mult4/1 -> Add4/1
  mult5/1 -> Add4/2
  [xd] -> mult4/2
  [xq] -> mult5/2
  [x0] -> Add4/3
  trigo/1 -> mult/1
  Gain1/1 -> mult1/1
  trigo2/1 -> mult2/1
  Gain2/1 -> mult3/1
  trigo4/1 -> mult4/1
  Gain3/1 -> mult5/1
  Add2/1 -> Mux/1  "xA"
  Add3/1 -> Mux/2  "xB"
  Add4/1 -> Mux/3  "xC"

== system ex14busSGandPV_sim/Photovoltaic Sources/measurements1 ==
  vdq0 : Inport
  idq0 : Inport  Port=2
  Add : Sum  Inputs=+++
  Add1 : Sum  Inputs=+-
  Add2 : Sum
  Demux : Demux  Outputs=3
  Demux1 : Demux  Outputs=3
  Gain : Gain  Gain=0.5
  Gain1 : Gain  Gain=0.5
  Gain2 : Gain  Gain=0.5
  Gain3 : Gain  Gain=2
  Gain4 : Gain  Gain=180/pi
  Math Function : Math  Operator=square  SaturateOnIntegerOverflow=on
  Math Function1 : Math  Operator=square  SaturateOnIntegerOverflow=on
  Sqrt : Sqrt  SaturateOnIntegerOverflow=on
  Trigonometric Function : Trigonometry  Operator=atan2
  mult{,1..4} (5 alike) : Product  Inputs=**
  P : Outport
  Q : Outport  Port=2
  Vm_RMS : Outport  Port=3
  Vph_deg : Outport  Port=4
  wires:
  idq0/1 -> Demux1/1
  vdq0/1 -> Demux/1
  Demux/1 -> Math Function/1, Trigonometric Function/2, mult3/1, mult/1  "vd"
  Demux/2 -> Trigonometric Function/1, Math Function1/1, mult2/1, mult1/1  "vq"
  Demux1/1 -> mult/2, mult2/2  "id"
  Demux1/2 -> mult3/2, mult1/2  "iq"
  Demux/3 -> mult4/1  "v0"
  Demux1/3 -> mult4/2  "i0"
  mult/1 -> Add/1
  mult1/1 -> Add/2
  Add/1 -> Gain/1
  mult2/1 -> Add1/1
  mult3/1 -> Add1/2
  Add1/1 -> Gain1/1
  Sqrt/1 -> Vm_RMS/1
  Math Function/1 -> Add2/1
  Math Function1/1 -> Add2/2
  Add2/1 -> Gain2/1
  Gain2/1 -> Sqrt/1
  Gain/1 -> P/1
  Gain1/1 -> Q/1
  mult4/1 -> Gain3/1
  Gain3/1 -> Add/3
  Trigonometric Function/1 -> Gain4/1
  Gain4/1 -> Vph_deg/1

== system ex14busSGandPV_sim/Photovoltaic Sources/measurements2 ==
  vdq0 : Inport
  idq0 : Inport  Port=2
  Add : Sum  Inputs=+++
  Add1 : Sum  Inputs=+-
  Add2 : Sum
  Demux : Demux  Outputs=3
  Demux1 : Demux  Outputs=3
  Gain : Gain  Gain=0.5
  Gain1 : Gain  Gain=0.5
  Gain2 : Gain  Gain=0.5
  Gain3 : Gain  Gain=2
  Gain4 : Gain  Gain=180/pi
  Math Function : Math  Operator=square  SaturateOnIntegerOverflow=on
  Math Function1 : Math  Operator=square  SaturateOnIntegerOverflow=on
  Sqrt : Sqrt  SaturateOnIntegerOverflow=on
  Trigonometric Function : Trigonometry  Operator=atan2
  mult{,1..4} (5 alike) : Product  Inputs=**
  P : Outport
  Q : Outport  Port=2
  Vm_RMS : Outport  Port=3
  Vph_deg : Outport  Port=4
  wires:
  idq0/1 -> Demux1/1
  vdq0/1 -> Demux/1
  Demux/1 -> Math Function/1, Trigonometric Function/2, mult3/1, mult/1  "vd"
  Demux/2 -> Trigonometric Function/1, Math Function1/1, mult2/1, mult1/1  "vq"
  Demux1/1 -> mult/2, mult2/2  "id"
  Demux1/2 -> mult3/2, mult1/2  "iq"
  Demux/3 -> mult4/1  "v0"
  Demux1/3 -> mult4/2  "i0"
  mult/1 -> Add/1
  mult1/1 -> Add/2
  Add/1 -> Gain/1
  mult2/1 -> Add1/1
  mult3/1 -> Add1/2
  Add1/1 -> Gain1/1
  Sqrt/1 -> Vm_RMS/1
  Math Function/1 -> Add2/1
  Math Function1/1 -> Add2/2
  Add2/1 -> Gain2/1
  Gain2/1 -> Sqrt/1
  Gain/1 -> P/1
  Gain1/1 -> Q/1
  mult4/1 -> Gain3/1
  Gain3/1 -> Add/3
  Trigonometric Function/1 -> Gain4/1
  Gain4/1 -> Vph_deg/1

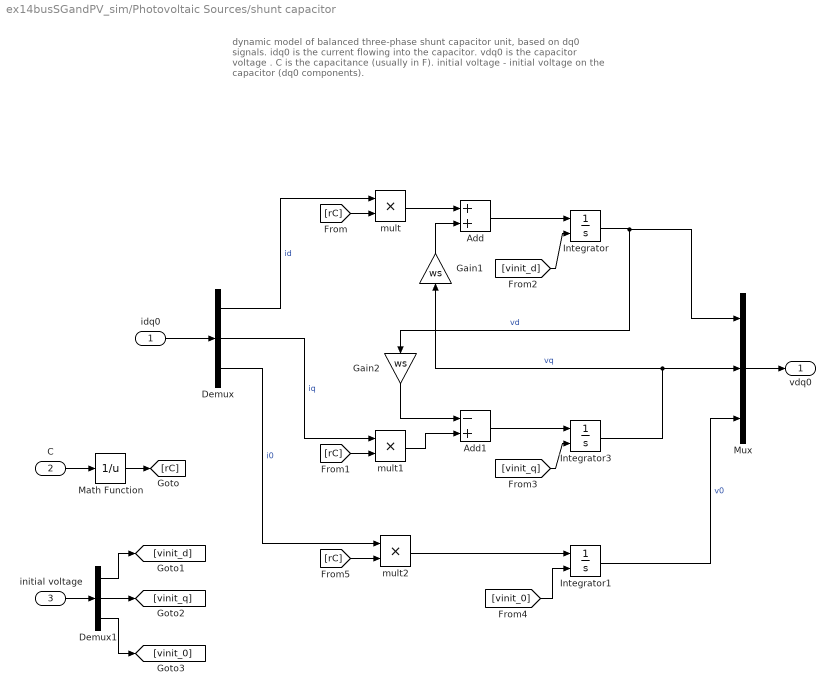
== system ex14busSGandPV_sim/Photovoltaic Sources/shunt capacitor ==
  note: dynamic model of balanced three-phase shunt capacitor unit, based on dq0 signals.
      | idq0 is the current flowing into the capacitor.
      | vdq0 is the capacitor voltage .
      | C is the capacitance (usually in F).
      | initial voltage - initial voltage on the capacitor (dq0 components).
  idq0 : Inport
  C : Inport  Port=2
  initial voltage : Inport  Port=3
  Add : Sum
  Add1 : Sum  Inputs=-+
  Demux : Demux  Outputs=3
  Demux1 : Demux  Outputs=3
  Gain1 : Gain  Gain=ws
  Gain2 : Gain  Gain=ws
  Integrator : Integrator  InitialConditionSource=external  InitialCondition=bus1_vd
  Integrator1 : Integrator  InitialConditionSource=external  InitialCondition=bus1_vd
  Integrator3 : Integrator  InitialConditionSource=external  InitialCondition=bus1_vd
  Math Function : Math  Operator=reciprocal  SaturateOnIntegerOverflow=on
  Mux : Mux  Inputs=3
  mult : Product  Inputs=**
  mult1 : Product  Inputs=**
  mult2 : Product  Inputs=**
  vdq0 : Outport
  wires:
  Integrator1/1 -> Mux/3  "v0"
  Mux/1 -> vdq0/1
  Integrator/1 -> Gain2/1, Mux/1  "vd"
  Integrator3/1 -> Gain1/1, Mux/2  "vq"
  Add/1 -> Integrator/1
  Gain1/1 -> Add/2
  idq0/1 -> Demux/1
  Demux/1 -> mult/1  "id"
  mult/1 -> Add/1
  Add1/1 -> Integrator3/1
  Gain2/1 -> Add1/1
  Demux/2 -> mult1/1  "iq"
  mult1/1 -> Add1/2
  Demux/3 -> mult2/1  "i0"
  mult2/1 -> Integrator1/1
  initial voltage/1 -> Demux1/1
  Demux1/1 -> [vinit_d]
  Demux1/2 -> [vinit_q]
  Demux1/3 -> [vinit_0]
  [vinit_d] -> Integrator/2
  [vinit_q] -> Integrator3/2
  [vinit_0] -> Integrator1/2
  C/1 -> Math Function/1
  Math Function/1 -> [rC]
  [rC] -> mult/2
  [rC] -> mult1/2
  [rC] -> mult2/2

== system ex14busSGandPV_sim/Photovoltaic Sources/shunt capacitor 1 ==
  note: dynamic model of balanced three-phase shunt capacitor unit, based on dq0 signals.
      | idq0 is the current flowing into the capacitor.
      | vdq0 is the capacitor voltage .
      | C is the capacitance (usually in F).
      | initial voltage - initial voltage on the capacitor (dq0 components).
  idq0 : Inport
  C : Inport  Port=2
  initial voltage : Inport  Port=3
  Add : Sum
  Add1 : Sum  Inputs=-+
  Demux : Demux  Outputs=3
  Demux1 : Demux  Outputs=3
  Gain1 : Gain  Gain=ws
  Gain2 : Gain  Gain=ws
  Integrator : Integrator  InitialConditionSource=external  InitialCondition=bus1_vd
  Integrator1 : Integrator  InitialConditionSource=external  InitialCondition=bus1_vd
  Integrator3 : Integrator  InitialConditionSource=external  InitialCondition=bus1_vd
  Math Function : Math  Operator=reciprocal  SaturateOnIntegerOverflow=on
  Mux : Mux  Inputs=3
  mult : Product  Inputs=**
  mult1 : Product  Inputs=**
  mult2 : Product  Inputs=**
  vdq0 : Outport
  wires:
  Integrator1/1 -> Mux/3  "v0"
  Mux/1 -> vdq0/1
  Integrator/1 -> Gain2/1, Mux/1  "vd"
  Integrator3/1 -> Gain1/1, Mux/2  "vq"
  Add/1 -> Integrator/1
  Gain1/1 -> Add/2
  idq0/1 -> Demux/1
  Demux/1 -> mult/1  "id"
  mult/1 -> Add/1
  Add1/1 -> Integrator3/1
  Gain2/1 -> Add1/1
  Demux/2 -> mult1/1  "iq"
  mult1/1 -> Add1/2
  Demux/3 -> mult2/1  "i0"
  mult2/1 -> Integrator1/1
  initial voltage/1 -> Demux1/1
  Demux1/1 -> [vinit_d]
  Demux1/2 -> [vinit_q]
  Demux1/3 -> [vinit_0]
  [vinit_d] -> Integrator/2
  [vinit_q] -> Integrator3/2
  [vinit_0] -> Integrator1/2
  C/1 -> Math Function/1
  Math Function/1 -> [rC]
  [rC] -> mult/2
  [rC] -> mult1/2
  [rC] -> mult2/2

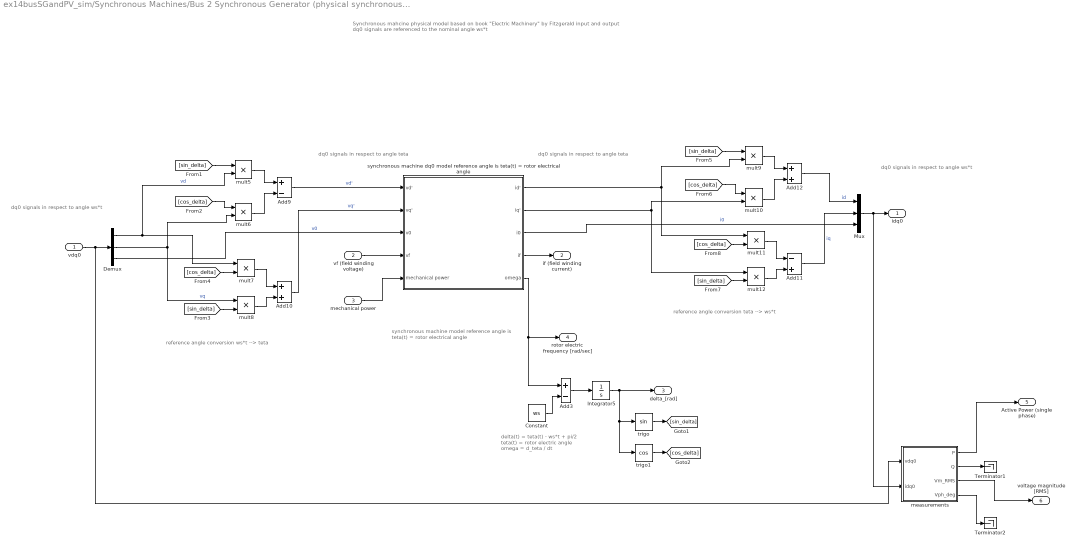
== system ex14busSGandPV_sim/Synchronous Machines/Bus 2 Synchronous Generator (physical synchronous machine model) ==
  note: Synchronous mahcine physical model
      | based on book "Electric Machinery" by Fitzgerald
      |
      | input and output dq0 signals are referenced
      | to the nominal angle ws*t
  note: reference angle conversion ws*t --> teta
  note: synchronous machine model
      | reference angle is
      | teta(t) = rotor electrical angle
  note: reference angle conversion teta --> ws*t
  note: dq0 signals in respect to angle ws*t
  note: dq0 signals in respect to angle ws*t
  note: dq0 signals in respect to angle teta
  note: dq0 signals in respect to angle teta
  note: delta(t) = teta(t) - ws*t + pi/2
      | teta(t) = rotor electric angle
      | omega = d_teta / dt
  vdq0 : Inport
  vf (field winding voltage) : Inport  Port=2
  mechanical power : Inport  Port=3
  Add10 : Sum
  Add11 : Sum  Inputs=-+
  Add12 : Sum
  Add3 : Sum  Inputs=+-
  Add9 : Sum  Inputs=+-
  Constant : Constant  Value=ws
  Demux : Demux  Outputs=3
  Integrator5 : Integrator
  Mux : Mux  Inputs=3
  Terminator1 : Terminator
  Terminator2 : Terminator
  measurements : Subsystem
  mult{5..12} (8 alike) : Product  Inputs=**
  synchronous machine dq0 model reference angle is teta(t) = rotor electrical angle : Subsystem
  trigo : Trigonometry
  trigo1 : Trigonometry  Operator=cos
  idq0 : Outport
  if (field winding current) : Outport  Port=2
  delta_[rad] : Outport  Port=3
  rotor electric frequency [rad/sec] : Outport  Port=4
  Active Power (single phase) : Outport  Port=5
  voltage magnitude [RMS] : Outport  Port=6
  wires:
  vdq0/1 -> measurements/1(vdq0), Demux/1
  Demux/1 -> mult5/2, mult7/1  "vd"
  Demux/2 -> mult6/2, mult8/1  "vq"
  mult5/1 -> Add9/1
  mult6/1 -> Add9/2
  [sin_delta] -> mult5/1
  [cos_delta] -> mult6/1
  mult7/1 -> Add10/1
  mult8/1 -> Add10/2
  [cos_delta] -> mult7/2
  [sin_delta] -> mult8/2
  mult9/1 -> Add12/1
  mult10/1 -> Add12/2
  [sin_delta] -> mult9/1
  [cos_delta] -> mult10/1
  mult11/1 -> Add11/1
  mult12/1 -> Add11/2
  [cos_delta] -> mult11/2
  [sin_delta] -> mult12/2
  Mux/1 -> measurements/2(idq0), idq0/1
  Add11/1 -> Mux/2  "iq"
  Add12/1 -> Mux/1  "id"
  synchronous machine dq0 model reference angle is teta(t) = rotor electrical angle/1(id') -> mult11/1, mult9/2
  synchronous machine dq0 model reference angle is teta(t) = rotor electrical angle/2(iq') -> mult12/1, mult10/2
  Add9/1 -> synchronous machine dq0 model reference angle is teta(t) = rotor electrical angle/1(vd')  "vd'"
  mechanical power/1 -> synchronous machine dq0 model reference angle is teta(t) = rotor electrical angle/5(mechanical power)
  Demux/3 -> synchronous machine dq0 model reference angle is teta(t) = rotor electrical angle/3(v0)  "v0"
  Add10/1 -> synchronous machine dq0 model reference angle is teta(t) = rotor electrical angle/2(vq')  "vq'"
  vf (field winding voltage)/1 -> synchronous machine dq0 model reference angle is teta(t) = rotor electrical angle/4(vf)
  synchronous machine dq0 model reference angle is teta(t) = rotor electrical angle/3(i0) -> Mux/3  "i0"
  synchronous machine dq0 model reference angle is teta(t) = rotor electrical angle/4(if) -> if (field winding current)/1
  trigo/1 -> [sin_delta]
  trigo1/1 -> [cos_delta]
  Add3/1 -> Integrator5/1
  Constant/1 -> Add3/2
  synchronous machine dq0 model reference angle is teta(t) = rotor electrical angle/5(omega) -> Add3/1, rotor electric frequency [rad/sec]/1
  Integrator5/1 -> delta_[rad]/1, trigo1/1, trigo/1
  measurements/1(P) -> Active Power (single phase)/1
  measurements/2(Q) -> Terminator1/1
  measurements/3(Vm_RMS) -> voltage magnitude [RMS]/1
  measurements/4(Vph_deg) -> Terminator2/1

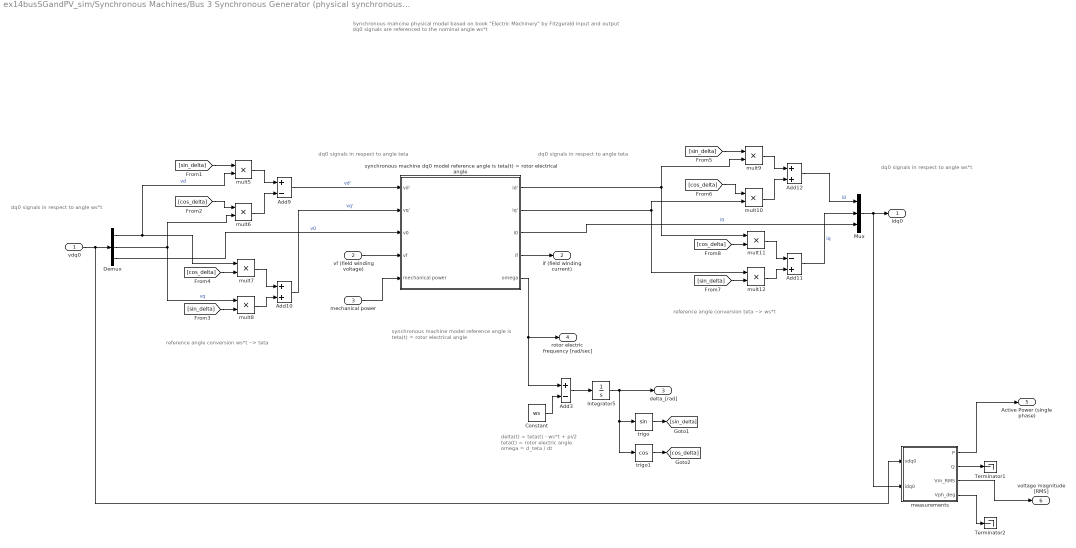
== system ex14busSGandPV_sim/Synchronous Machines/Bus 3 Synchronous Generator (physical synchronous machine model) ==
  note: Synchronous mahcine physical model
      | based on book "Electric Machinery" by Fitzgerald
      |
      | input and output dq0 signals are referenced
      | to the nominal angle ws*t
  note: reference angle conversion ws*t --> teta
  note: synchronous machine model
      | reference angle is
      | teta(t) = rotor electrical angle
  note: reference angle conversion teta --> ws*t
  note: dq0 signals in respect to angle ws*t
  note: dq0 signals in respect to angle ws*t
  note: dq0 signals in respect to angle teta
  note: dq0 signals in respect to angle teta
  note: delta(t) = teta(t) - ws*t + pi/2
      | teta(t) = rotor electric angle
      | omega = d_teta / dt
  vdq0 : Inport
  vf (field winding voltage) : Inport  Port=2
  mechanical power : Inport  Port=3
  Add10 : Sum
  Add11 : Sum  Inputs=-+
  Add12 : Sum
  Add3 : Sum  Inputs=+-
  Add9 : Sum  Inputs=+-
  Constant : Constant  Value=ws
  Demux : Demux  Outputs=3
  Integrator5 : Integrator
  Mux : Mux  Inputs=3
  Terminator1 : Terminator
  Terminator2 : Terminator
  measurements : Subsystem
  mult{5..12} (8 alike) : Product  Inputs=**
  synchronous machine dq0 model reference angle is teta(t) = rotor electrical angle : Subsystem
  trigo : Trigonometry
  trigo1 : Trigonometry  Operator=cos
  idq0 : Outport
  if (field winding current) : Outport  Port=2
  delta_[rad] : Outport  Port=3
  rotor electric frequency [rad/sec] : Outport  Port=4
  Active Power (single phase) : Outport  Port=5
  voltage magnitude [RMS] : Outport  Port=6
  wires:
  vdq0/1 -> measurements/1(vdq0), Demux/1
  Demux/1 -> mult5/2, mult7/1  "vd"
  Demux/2 -> mult6/2, mult8/1  "vq"
  mult5/1 -> Add9/1
  mult6/1 -> Add9/2
  [sin_delta] -> mult5/1
  [cos_delta] -> mult6/1
  mult7/1 -> Add10/1
  mult8/1 -> Add10/2
  [cos_delta] -> mult7/2
  [sin_delta] -> mult8/2
  mult9/1 -> Add12/1
  mult10/1 -> Add12/2
  [sin_delta] -> mult9/1
  [cos_delta] -> mult10/1
  mult11/1 -> Add11/1
  mult12/1 -> Add11/2
  [cos_delta] -> mult11/2
  [sin_delta] -> mult12/2
  Mux/1 -> measurements/2(idq0), idq0/1
  Add11/1 -> Mux/2  "iq"
  Add12/1 -> Mux/1  "id"
  synchronous machine dq0 model reference angle is teta(t) = rotor electrical angle/1(id') -> mult11/1, mult9/2
  synchronous machine dq0 model reference angle is teta(t) = rotor electrical angle/2(iq') -> mult12/1, mult10/2
  Add9/1 -> synchronous machine dq0 model reference angle is teta(t) = rotor electrical angle/1(vd')  "vd'"
  mechanical power/1 -> synchronous machine dq0 model reference angle is teta(t) = rotor electrical angle/5(mechanical power)
  Demux/3 -> synchronous machine dq0 model reference angle is teta(t) = rotor electrical angle/3(v0)  "v0"
  Add10/1 -> synchronous machine dq0 model reference angle is teta(t) = rotor electrical angle/2(vq')  "vq'"
  vf (field winding voltage)/1 -> synchronous machine dq0 model reference angle is teta(t) = rotor electrical angle/4(vf)
  synchronous machine dq0 model reference angle is teta(t) = rotor electrical angle/3(i0) -> Mux/3  "i0"
  synchronous machine dq0 model reference angle is teta(t) = rotor electrical angle/4(if) -> if (field winding current)/1
  trigo/1 -> [sin_delta]
  trigo1/1 -> [cos_delta]
  Add3/1 -> Integrator5/1
  Constant/1 -> Add3/2
  synchronous machine dq0 model reference angle is teta(t) = rotor electrical angle/5(omega) -> Add3/1, rotor electric frequency [rad/sec]/1
  Integrator5/1 -> delta_[rad]/1, trigo1/1, trigo/1
  measurements/1(P) -> Active Power (single phase)/1
  measurements/2(Q) -> Terminator1/1
  measurements/3(Vm_RMS) -> voltage magnitude [RMS]/1
  measurements/4(Vph_deg) -> Terminator2/1

== system ex14busSGandPV_sim/Synchronous Machines/shunt capacitor 2 ==
  note: dynamic model of balanced three-phase shunt capacitor unit, based on dq0 signals.
      | idq0 is the current flowing into the capacitor.
      | vdq0 is the capacitor voltage .
      | C is the capacitance (usually in F).
      | initial voltage - initial voltage on the capacitor (dq0 components).
  idq0 : Inport
  C : Inport  Port=2
  initial voltage : Inport  Port=3
  Add : Sum
  Add1 : Sum  Inputs=-+
  Demux : Demux  Outputs=3
  Demux1 : Demux  Outputs=3
  Gain1 : Gain  Gain=ws
  Gain2 : Gain  Gain=ws
  Integrator : Integrator  InitialConditionSource=external  InitialCondition=bus1_vd
  Integrator1 : Integrator  InitialConditionSource=external  InitialCondition=bus1_vd
  Integrator3 : Integrator  InitialConditionSource=external  InitialCondition=bus1_vd
  Math Function : Math  Operator=reciprocal  SaturateOnIntegerOverflow=on
  Mux : Mux  Inputs=3
  mult : Product  Inputs=**
  mult1 : Product  Inputs=**
  mult2 : Product  Inputs=**
  vdq0 : Outport
  wires:
  Integrator1/1 -> Mux/3  "v0"
  Mux/1 -> vdq0/1
  Integrator/1 -> Gain2/1, Mux/1  "vd"
  Integrator3/1 -> Gain1/1, Mux/2  "vq"
  Add/1 -> Integrator/1
  Gain1/1 -> Add/2
  idq0/1 -> Demux/1
  Demux/1 -> mult/1  "id"
  mult/1 -> Add/1
  Add1/1 -> Integrator3/1
  Gain2/1 -> Add1/1
  Demux/2 -> mult1/1  "iq"
  mult1/1 -> Add1/2
  Demux/3 -> mult2/1  "i0"
  mult2/1 -> Integrator1/1
  initial voltage/1 -> Demux1/1
  Demux1/1 -> [vinit_d]
  Demux1/2 -> [vinit_q]
  Demux1/3 -> [vinit_0]
  [vinit_d] -> Integrator/2
  [vinit_q] -> Integrator3/2
  [vinit_0] -> Integrator1/2
  C/1 -> Math Function/1
  Math Function/1 -> [rC]
  [rC] -> mult/2
  [rC] -> mult1/2
  [rC] -> mult2/2

== system ex14busSGandPV_sim/Synchronous Machines/shunt capacitor 3 ==
  note: dynamic model of balanced three-phase shunt capacitor unit, based on dq0 signals.
      | idq0 is the current flowing into the capacitor.
      | vdq0 is the capacitor voltage .
      | C is the capacitance (usually in F).
      | initial voltage - initial voltage on the capacitor (dq0 components).
  idq0 : Inport
  C : Inport  Port=2
  initial voltage : Inport  Port=3
  Add : Sum
  Add1 : Sum  Inputs=-+
  Demux : Demux  Outputs=3
  Demux1 : Demux  Outputs=3
  Gain1 : Gain  Gain=ws
  Gain2 : Gain  Gain=ws
  Integrator : Integrator  InitialConditionSource=external  InitialCondition=bus1_vd
  Integrator1 : Integrator  InitialConditionSource=external  InitialCondition=bus1_vd
  Integrator3 : Integrator  InitialConditionSource=external  InitialCondition=bus1_vd
  Math Function : Math  Operator=reciprocal  SaturateOnIntegerOverflow=on
  Mux : Mux  Inputs=3
  mult : Product  Inputs=**
  mult1 : Product  Inputs=**
  mult2 : Product  Inputs=**
  vdq0 : Outport
  wires:
  Integrator1/1 -> Mux/3  "v0"
  Mux/1 -> vdq0/1
  Integrator/1 -> Gain2/1, Mux/1  "vd"
  Integrator3/1 -> Gain1/1, Mux/2  "vq"
  Add/1 -> Integrator/1
  Gain1/1 -> Add/2
  idq0/1 -> Demux/1
  Demux/1 -> mult/1  "id"
  mult/1 -> Add/1
  Add1/1 -> Integrator3/1
  Gain2/1 -> Add1/1
  Demux/2 -> mult1/1  "iq"
  mult1/1 -> Add1/2
  Demux/3 -> mult2/1  "i0"
  mult2/1 -> Integrator1/1
  initial voltage/1 -> Demux1/1
  Demux1/1 -> [vinit_d]
  Demux1/2 -> [vinit_q]
  Demux1/3 -> [vinit_0]
  [vinit_d] -> Integrator/2
  [vinit_q] -> Integrator3/2
  [vinit_0] -> Integrator1/2
  C/1 -> Math Function/1
  Math Function/1 -> [rC]
  [rC] -> mult/2
  [rC] -> mult1/2
  [rC] -> mult2/2

== system ex14busSGandPV_sim/Synchronous Machines/Bus 2 Synchronous Generator (physical synchronous machine model)/measurements ==
  vdq0 : Inport
  idq0 : Inport  Port=2
  Add : Sum  Inputs=+++
  Add1 : Sum  Inputs=+-
  Add2 : Sum
  Demux : Demux  Outputs=3
  Demux1 : Demux  Outputs=3
  Gain : Gain  Gain=0.5
  Gain1 : Gain  Gain=0.5
  Gain2 : Gain  Gain=0.5
  Gain3 : Gain  Gain=2
  Gain4 : Gain  Gain=180/pi
  Math Function : Math  Operator=square  SaturateOnIntegerOverflow=on
  Math Function1 : Math  Operator=square  SaturateOnIntegerOverflow=on
  Sqrt : Sqrt  SaturateOnIntegerOverflow=on
  Trigonometric Function : Trigonometry  Operator=atan2
  mult{,1..4} (5 alike) : Product  Inputs=**
  P : Outport
  Q : Outport  Port=2
  Vm_RMS : Outport  Port=3
  Vph_deg : Outport  Port=4
  wires:
  idq0/1 -> Demux1/1
  vdq0/1 -> Demux/1
  Demux/1 -> Math Function/1, Trigonometric Function/2, mult3/1, mult/1  "vd"
  Demux/2 -> Trigonometric Function/1, Math Function1/1, mult2/1, mult1/1  "vq"
  Demux1/1 -> mult/2, mult2/2  "id"
  Demux1/2 -> mult3/2, mult1/2  "iq"
  Demux/3 -> mult4/1  "v0"
  Demux1/3 -> mult4/2  "i0"
  mult/1 -> Add/1
  mult1/1 -> Add/2
  Add/1 -> Gain/1
  mult2/1 -> Add1/1
  mult3/1 -> Add1/2
  Add1/1 -> Gain1/1
  Sqrt/1 -> Vm_RMS/1
  Math Function/1 -> Add2/1
  Math Function1/1 -> Add2/2
  Add2/1 -> Gain2/1
  Gain2/1 -> Sqrt/1
  Gain/1 -> P/1
  Gain1/1 -> Q/1
  mult4/1 -> Gain3/1
  Gain3/1 -> Add/3
  Trigonometric Function/1 -> Gain4/1
  Gain4/1 -> Vph_deg/1
